simulink model "cool_model_1"  (Simulink 8.3)
settings: Solver=ode45  StartTime=0.0  StopTime=20.0  RelTol=1e-3
settings Model: Creator=stud507ikt  LastModifiedBy=stud507ikt
settings DataIOCC: SignalLoggingSaveFormat=Dataset
settings DebuggingCC: UnderspecifiedInitializationDetection=Simplified  StateNameClashWarn=none
settings GRTTargetCC: CombineOutputUpdateFcns=on  GRTInterface=off

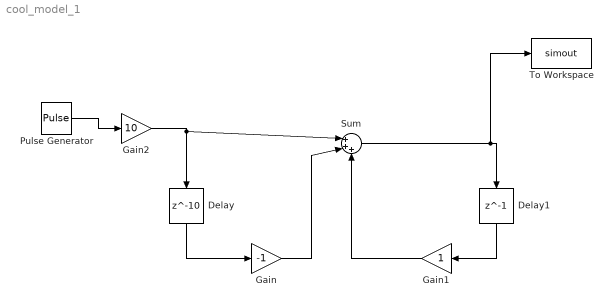
== system cool_model_1 ==
  Delay : Delay  DelayLength=10  InitialCondition=0  InputProcessing=Inherited
  Delay1 : Delay  DelayLength=1  InitialCondition=0  InputProcessing=Inherited
  Gain : Gain  Gain=-1
  Gain1 : Gain
  Gain2 : Gain  Gain=10
  Pulse Generator : DiscretePulseGenerator  Period=100
  Sum : Sum  Inputs=|+++
  To Workspace : ToWorkspace  VariableName=simout  SampleTime=-1
  wires:
  Gain1/1 -> Sum/3
  Delay1/1 -> Gain1/1
  Sum/1 -> To Workspace/1, Delay1/1
  Gain/1 -> Sum/2
  Delay/1 -> Gain/1
  Pulse Generator/1 -> Gain2/1
  Gain2/1 -> Delay/1, Sum/1
